simulink subsystem "NoThermalEffectSSC"  (R2024a)
settings: Solver=VariableStepAuto  StartTime=0.0  StopTime=10.0  RelTol=1e-3
undefined symbols (not defined in the file): EnvAirTemp, ThrmBatt1, ThrmBatt2, ThrmBatt3, ThrmBatt4, ThrmEM1, ThrmEM2, ThrmEM3, ThrmEM4
libraries: fl_lib x9
settings Model: ModifiedByFormat=The MathWorks, Inc.  Creator=The MathWorks, Inc.  LastModifiedBy=The MathWorks, Inc.
settings DebuggingCC: SubsystemReferenceDiagnosticForUnitTest=warning
settings RTWCC: GPUComputeCapability=3.5  LargeConstantGeneration=WriteOnlyDNNConstantsToDataFiles

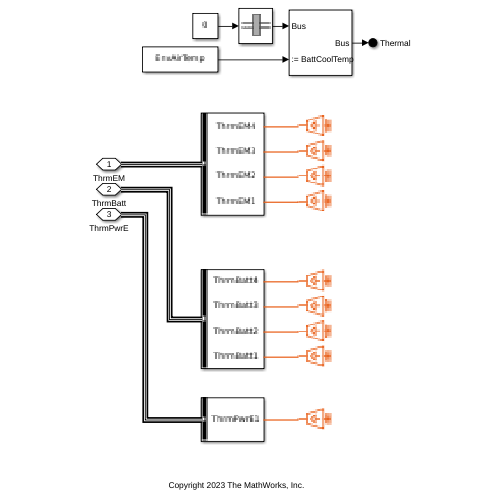
[thumbnail: Simulink's stored preview of the top-level diagram]
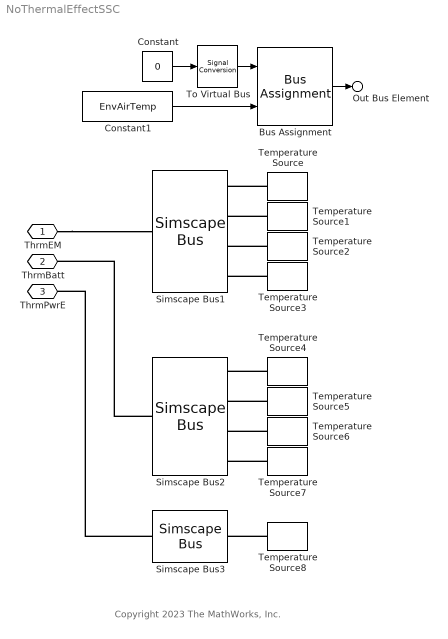
== system NoThermalEffectSSC ==
  note: Copyright 2023 The MathWorks, Inc.
  Bus Assignment : BusAssignment  AssignedSignals=BattCoolTemp
  Constant : Constant  Value=0  OutDataTypeStr=Bus: ThermalBUS  SampleTime=-1
  Constant1 : Constant  Value=EnvAirTemp  SampleTime=-1
  Simscape Bus1 : SimscapeBus  HierarchyStrings=ThrmEM4;ThrmEM3;ThrmEM2;ThrmEM1
  Simscape Bus2 : SimscapeBus  HierarchyStrings=ThrmBatt4;ThrmBatt3;ThrmBatt2;ThrmBatt1
  Simscape Bus3 : SimscapeBus  HierarchyStrings=ThrmPwrE1
  Temperature Source{,1..8} (9 alike) : fl_lib/Thermal/Thermal Sources/Temperature Source  temperature=EnvAirTemp K
  To Virtual Bus : SignalConversion  ConversionOutput=Virtual bus  OverrideOpt=off
  ThrmEM : PMIOPort  Side=Left
  ThrmBatt : PMIOPort  Port=2  Side=Left
  ThrmPwrE : PMIOPort  Port=3  Side=Left
  Out Bus Element : Outport  PortName=Thermal
  wires:
  Constant/1 -> To Virtual Bus/1
  Bus Assignment/1 -> Out Bus Element/1
  Constant1/1 -> Bus Assignment/2
  To Virtual Bus/1 -> Bus Assignment/1
  connections:
  Temperature Source8/LConn1 -- Simscape Bus3/LConn1
  Temperature Source2/LConn1 -- Simscape Bus1/LConn3
  Simscape Bus3/RConn1 -- ThrmPwrE/RConn1
  ThrmEM/RConn1 -- Simscape Bus1/RConn1
  Temperature Source/LConn1 -- Simscape Bus1/LConn1
  Temperature Source1/LConn1 -- Simscape Bus1/LConn2
  Simscape Bus2/RConn1 -- ThrmBatt/RConn1
  Temperature Source3/LConn1 -- Simscape Bus1/LConn4
  Temperature Source6/LConn1 -- Simscape Bus2/LConn3
  Temperature Source7/LConn1 -- Simscape Bus2/LConn4
  Temperature Source5/LConn1 -- Simscape Bus2/LConn2
  Temperature Source4/LConn1 -- Simscape Bus2/LConn1
